simulink model "RaketenMolell_V1"  (R2021b)
settings: Solver=VariableStepAuto  StartTime=0.0  StopTime=20.0  RelTol=1e-3
settings Model: VariantFading=off  Creator=tim  LastModifiedBy=tim

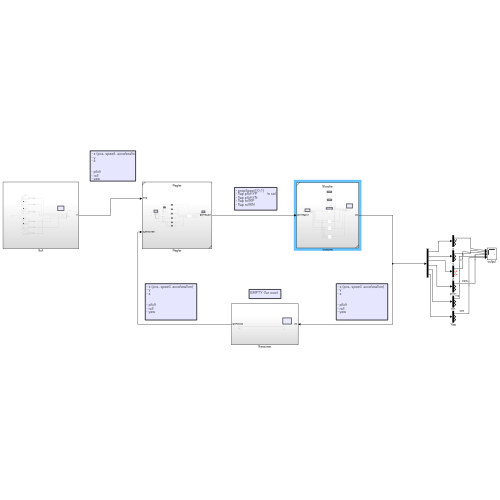
[thumbnail: Simulink's stored preview of the top-level diagram]
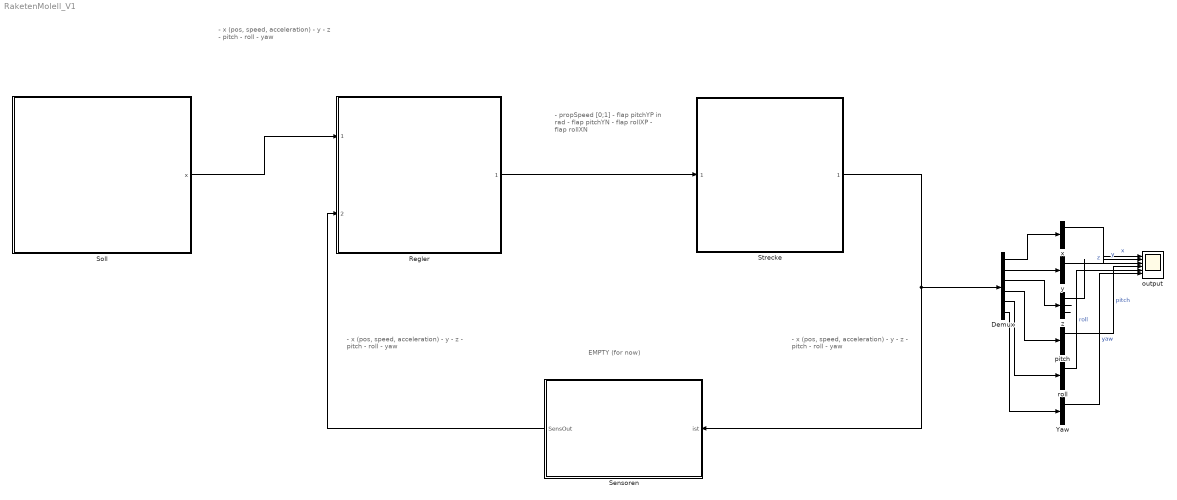
== system RaketenMolell_V1 ==
  note: EMPTY (for now)
  note: - x (pos, speed, acceleration)
      | - y
      | - z
      |
      |
      | - pitch
      | - roll
      | - yaw
  note: - x (pos, speed, acceleration)
      | - y
      | - z
      |
      |
      | - pitch
      | - roll
      | - yaw
  note: - x (pos, speed, acceleration)
      | - y
      | - z
      |
      |
      | - pitch
      | - roll
      | - yaw
  note: - propSpeed [0;1]
      | - flap pitchYP          in rad
      | - flap pitchYN
      | - flap rollXP
      | - flap rollXN
  Demux : Demux  Outputs=[3 3 3 3 3 3]
  Regler : Subsystem  VariantControl=Choice  ReferencedSubsystem=Regler
  Sensoren : Subsystem
      settings: PortSchema="{\"entries\":[{\"content\":{\"sides\":[{\"content\":{\"connectorIds\":[\"Out1\"]},\"type\":\"ConnectorPlacement.EquallySpacedRectSide\",\"uuid\":\"1d466140-1e55-44c9-9bcb-efad05c0ea40\"},{\"content\":{\"connectorIds\":[\"In1\"],\"side\":\"RIGHT\"},\"type\":\"ConnectorPlacement.EquallySpacedRectSide\",\"uuid\":\"5a663876-4ac4-465d-b352-113c7e4c8b4d\"},{\"content\":{\"connectorIds\":[],\"side\":\"TOP\"},\"type\":\"ConnectorPlacement.EquallySpacedRectSide\",\"uuid\":\"b7c3ee67-cad3-4a04-95b6-95c30c2ee550\"}]},\"type\":\"ConnectorPlacement.EquallySpacedConnector\",\"uuid\":\"cf49840c-5e92-4b13-9a85-54e5cf2cde79\"}],\"packageUris\":[\"http://schema.mathworks.com/mf0/Connector/R2020b\"],\"version\":\"1.0\"}"
  Soll : Subsystem
  Strecke : Subsystem  ReferencedSubsystem=Strecke
  Yaw : Demux  Outputs=3
  output : Scope  NumInputPorts=6
  pitch : Demux  Outputs=3
  roll : Demux  Outputs=3
  x : Demux  Outputs=3
  y : Demux  Outputs=3
  z : Demux  Outputs=3
  wires:
  Strecke/1 -> Demux/1, Sensoren/1(ist)
  x/1 -> output/1  "x"
  Demux/1 -> x/1
  Demux/3 -> z/1
  y/1 -> output/2  "y"
  Demux/2 -> y/1
  Demux/4 -> pitch/1
  Demux/5 -> roll/1
  Demux/6 -> Yaw/1
  z/1 -> output/3  "z"
  pitch/1 -> output/4  "pitch"
  roll/1 -> output/5  "roll"
  Yaw/1 -> output/6  "yaw"
  Soll/1(x) -> Regler/1
  Sensoren/1(SensOut) -> Regler/2
  Regler/1 -> Strecke/1
  z/2 -> ?
  z/3 -> ?

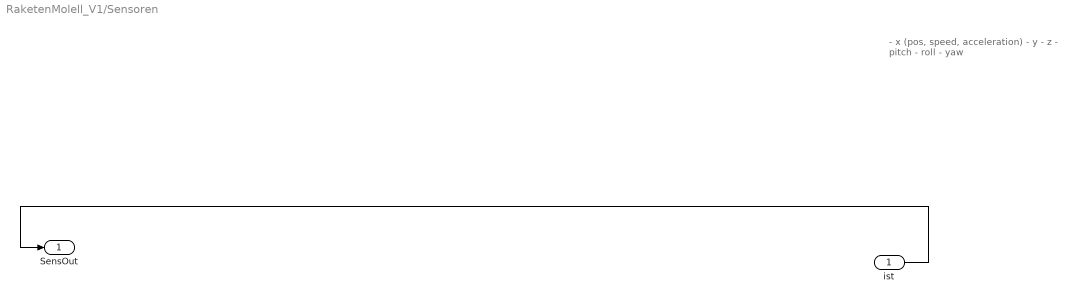
== system RaketenMolell_V1/Sensoren ==
  note: - x (pos, speed, acceleration)
      | - y
      | - z
      |
      |
      | - pitch
      | - roll
      | - yaw
  ist : Inport
  SensOut : Outport
  wires:
  ist/1 -> SensOut/1

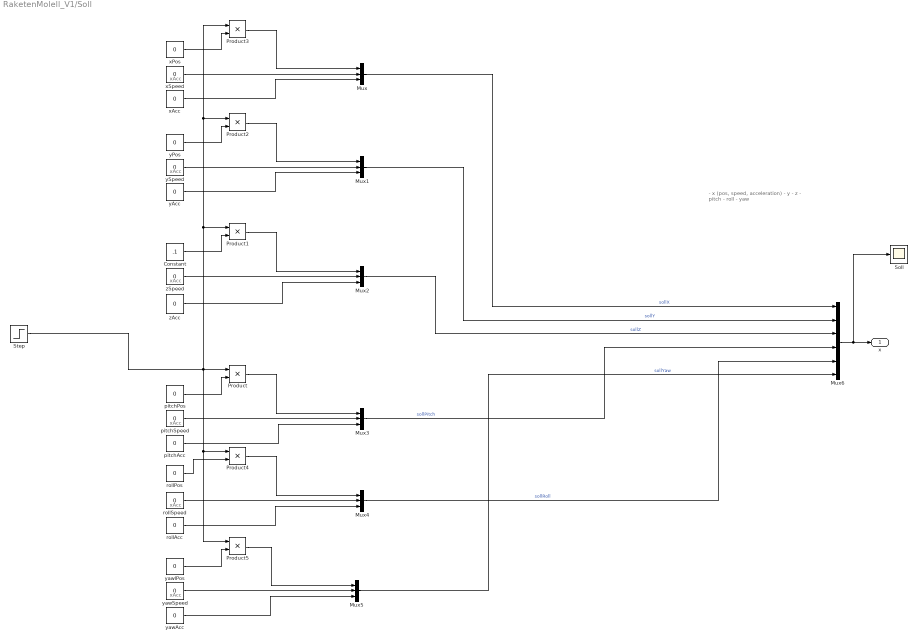
== system RaketenMolell_V1/Soll ==
  note: - x (pos, speed, acceleration)
      | - y
      | - z
      |
      |
      | - pitch
      | - roll
      | - yaw
  note: xAcc
  note: xAcc
  note: xAcc
  note: xAcc
  note: xAcc
  note: xAcc
  Constant : Constant  Value=.1
  Mux{,1..5} (6 alike) : Mux  Inputs=3
  Mux6 : Mux  Inputs=6
  Product{,1..5} (6 alike) : Product
  Soll : Scope
  Step : Step  SampleTime=0
  pitchAcc : Constant  Value=0
  pitchPos : Constant  Value=0
  pitchSpeed : Constant  Value=0
  rollAcc : Constant  Value=0
  rollPos : Constant  Value=0
  rollSpeed : Constant  Value=0
  xAcc : Constant  Value=0
  xPos : Constant  Value=0
  xSpeed : Constant  Value=0
  yAcc : Constant  Value=0
  yPos : Constant  Value=0
  ySpeed : Constant  Value=0
  yawAcc : Constant  Value=0
  yawSpeed : Constant  Value=0
  yawlPos : Constant  Value=0
  zAcc : Constant  Value=0
  zSpeed : Constant  Value=0
  x : Outport
  wires:
  Mux/1 -> Mux6/1  "sollX"
  Mux1/1 -> Mux6/2  "sollY"
  Mux2/1 -> Mux6/3  "sollZ"
  Mux4/1 -> Mux6/5  "sollRoll"
  Mux5/1 -> Mux6/6  "sollYaw"
  Mux3/1 -> Mux6/4  "sollPitch"
  Mux6/1 -> Soll/1, x/1
  pitchAcc/1 -> Mux3/3
  pitchSpeed/1 -> Mux3/2
  Product/1 -> Mux3/1
  pitchPos/1 -> Product/2
  zAcc/1 -> Mux2/3
  zSpeed/1 -> Mux2/2
  Product1/1 -> Mux2/1
  Constant/1 -> Product1/2
  yAcc/1 -> Mux1/3
  ySpeed/1 -> Mux1/2
  Product2/1 -> Mux1/1
  yPos/1 -> Product2/2
  xAcc/1 -> Mux/3
  xSpeed/1 -> Mux/2
  Product3/1 -> Mux/1
  xPos/1 -> Product3/2
  rollAcc/1 -> Mux4/3
  rollSpeed/1 -> Mux4/2
  Product4/1 -> Mux4/1
  rollPos/1 -> Product4/2
  yawlPos/1 -> Product5/2
  yawSpeed/1 -> Mux5/2
  yawAcc/1 -> Mux5/3
  Product5/1 -> Mux5/1
  Step/1 -> Product3/1, Product2/1, Product1/1, Product5/1, Product4/1, Product/1
